simulink model "tracked_robot"  (R2023a)
settings: Solver=FixedStepDiscrete  StartTime=0.0  StopTime=sim_param.t_end  FixedStep=sim_param.dt  RelTol=1e-3  EnableMultiTasking=on
InitFcn:
  | initfcn
values from neighbouring files (symbols this model uses):
  slip_compensation = 1    [plots.m]    (also in tracked_robot_param.m = 0)
undefined symbols (not defined in the file or in its folder): DiscIntNeverNeededParam, param, path_param, sim_param
libraries: simulink x2
settings Model: PacingRate=0.002500  Creator=david  LastModifiedBy=mfocchi
settings SolverCC: AutoInsertRateTranBlk=on
settings OptimizationCC: DefaultParameterBehavior=Inlined  UseDivisionForNetSlopeComputation=on  GainParamInheritBuiltInType=on  UseFloatMulNetSlope=on  InlineInvariantSignals=on  PassReuseOutputArgsAs=Individual arguments  ZeroExternalMemoryAtStartup=off  ZeroInternalMemoryAtStartup=off  NoFixptDivByZeroProtection=on  EfficientFloat2IntCast=on  LifeSpan=1  OptimizeBlockOrder=speed  DifferentSizesBufferReuse=on  EfficientTunableParamExpr=on
settings DebuggingCC: ParameterTunabilityLossMsg=error  UnderSpecifiedDimensionMsg=warning
settings HardwareCC: ProdLongLongMode=on
settings ModelReferenceCC: ModelReferenceMinAlgLoopOccurrences=on
settings SFSimCC: MATLABDynamicMemAlloc=off
settings RTWCC: Description=Embedded Coder  SystemTargetFile=ert.tlc  TemplateMakefile=ert_default_tmf  TargetLang=C++
settings CodeAppCC: ForceParamTrailComments=on  IgnoreCustomStorageClasses=off  OperatorAnnotations=on  SimulinkDataObjDesc=on  SFDataObjDesc=on  CustomSymbolStrGlobalVar=rt$N$M  CustomSymbolStrType=$N$M  CustomSymbolStrFcn=$N$M$F  CustomSymbolStrMacro=$N$M  InsertBlockDesc=on
settings ERTTargetCC: TargetLangStandard=C++11 (ISO)  GenerateSampleERTMain=on  IncludeMdlTerminateFcn=off  CombineSignalStateStructs=on  CodeInterfacePackaging=C++ class  SupportComplex=off  SupportContinuousTime=on  SupportNonInlinedSFcns=on  SupportVariableSizeSignals=on  InlinedParameterPlacement=NonHierarchical  RootIOFormat=Structure reference  ERTCustomFileTemplate=example_file_process.tlc  ERTFilePackagingFormat=CompactWithDataFile

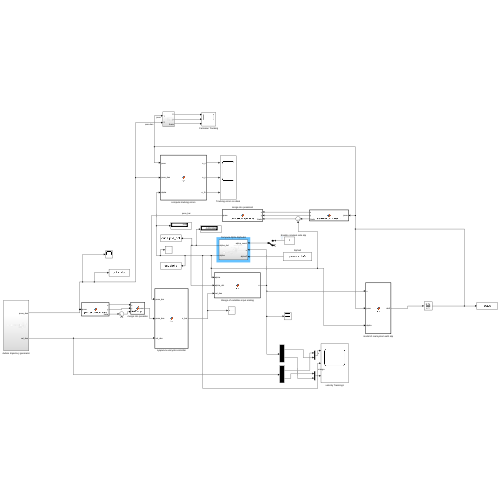
[thumbnail: Simulink's stored preview of the top-level diagram]
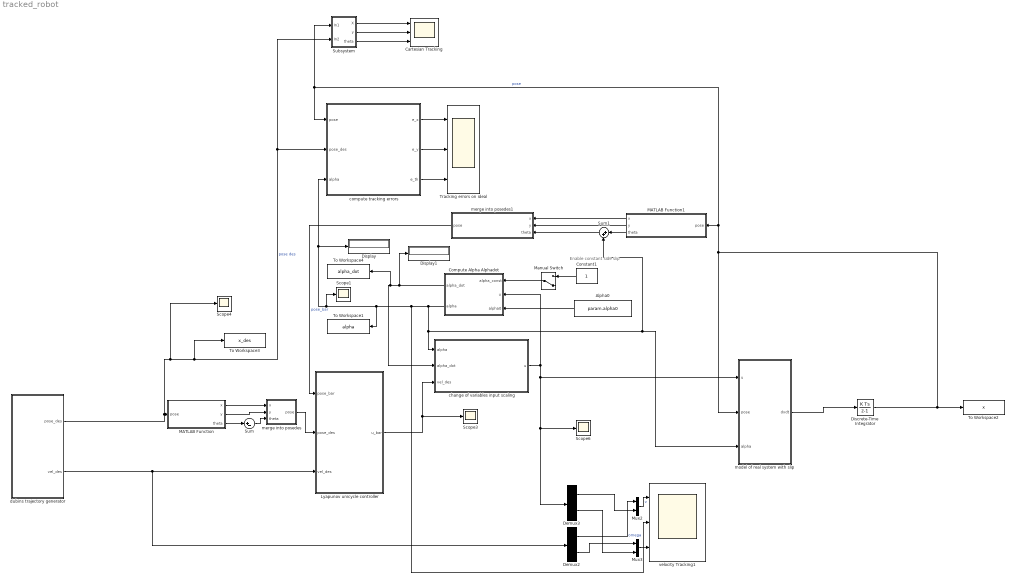
== system tracked_robot ==
  note: Enable constant side slip
  Alpha0 : Constant  Value=param.alpha0
  Cartesian Tracking : Scope  NumInputPorts=3
  Compute Alpha Alphadot : Subsystem
  Constant1 : Constant
  Demux2 : Demux  Outputs=2
  Demux3 : Demux  Outputs=2
  Discrete-Time Integrator : DiscreteIntegrator  InitialCondition=sim_param.initial_state  SampleTime=sim_param.dt  ICPrevOutput=DiscIntNeverNeededParam  ICPrevScaledInput=DiscIntNeverNeededParam
  Display : Display
  Display1 : Display
  Lyapunov unicycle controller : MATLAB Function  TreatAsAtomicUnit=on
  MATLAB Function : MATLAB Function  TreatAsAtomicUnit=on
  MATLAB Function1 : MATLAB Function  TreatAsAtomicUnit=on
  Manual Switch : ManualSwitch  CurrentSetting=0
  Mux2 : Mux  Inputs=2
  Mux3 : Mux  Inputs=2
  Scope{1,3..4,6} (4 alike) : Scope
  Subsystem : Subsystem
  Sum : Sum  Inputs=|+-
  Sum1 : Sum  Inputs=|++
  To Workspace1 : ToWorkspace  VariableName=alpha  SaveFormat=Timeseries  SampleTime=-1
      settings: Decimation=sim_param.decimation
  To Workspace2 : ToWorkspace  VariableName=x  SaveFormat=Timeseries  SampleTime=-1
      settings: Decimation=sim_param.decimation
  To Workspace3 : ToWorkspace  VariableName=x_des  SaveFormat=Timeseries  SampleTime=-1
      settings: Decimation=sim_param.decimation
  To Workspace4 : ToWorkspace  VariableName=alpha_dot  SaveFormat=Timeseries  SampleTime=-1
      settings: Decimation=sim_param.decimation
  Tracking errors on ideal : Scope  NumInputPorts=3
  change of variables input scaling : MATLAB Function  TreatAsAtomicUnit=on
  compute tracking errors : MATLAB Function  TreatAsAtomicUnit=on
  dubins trajectory generator : Subsystem
  merge into posedes : MATLAB Function  TreatAsAtomicUnit=on
  merge into posedes1 : MATLAB Function  TreatAsAtomicUnit=on
  model of real system with slip : MATLAB Function  TreatAsAtomicUnit=on
  velocity Tracking1 : Scope  NumInputPorts=3
  wires:
  model of real system with slip/1(dxdt) -> Discrete-Time Integrator/1
  dubins trajectory generator/1(pose_des) -> Subsystem/2(In2), compute tracking errors/2(pose_des), To Workspace3/1, Scope4/1, MATLAB Function/1(pose)  "pose des"
  Discrete-Time Integrator/1 -> To Workspace2/1, MATLAB Function1/1(pose), Subsystem/1(In1), compute tracking errors/1(pose), model of real system with slip/2(pose)  "pose"
  Lyapunov unicycle controller/1(u_bar) -> Scope3/1, change of variables input scaling/3(vel_des)
  MATLAB Function/1(x) -> merge into posedes/1(x)
  MATLAB Function/2(y) -> merge into posedes/2(y)
  MATLAB Function/3(theta) -> Sum/1
  Sum/1 -> merge into posedes/3(theta)
  merge into posedes/1(pose) -> Lyapunov unicycle controller/2(pose_des)
  compute tracking errors/1(e_x) -> Tracking errors on ideal/1
  compute tracking errors/2(e_y) -> Tracking errors on ideal/2
  compute tracking errors/3(e_th) -> Tracking errors on ideal/3
  Alpha0/1 -> Compute Alpha Alphadot/3(alpha0)
  Compute Alpha Alphadot/1(alpha_dot) -> To Workspace4/1, change of variables input scaling/2(alpha_dot), Display1/1
  Mux2/1 -> velocity Tracking1/1  "v"
  Mux3/1 -> velocity Tracking1/2  "omega"
  dubins trajectory generator/2(vel_des) -> Demux2/1, Lyapunov unicycle controller/3(vel_des)
  Demux2/1 -> Mux2/1
  Demux2/2 -> Mux3/1
  Demux3/1 -> Mux2/2
  Demux3/2 -> Mux3/2
  Constant1/1 -> Manual Switch/1
  Manual Switch/1 -> Compute Alpha Alphadot/1(alpha_const)
  MATLAB Function1/1(x) -> merge into posedes1/1(x)
  MATLAB Function1/2(y) -> merge into posedes1/2(y)
  Sum1/1 -> merge into posedes1/3(theta)
  MATLAB Function1/3(theta) -> Sum1/1
  merge into posedes1/1(pose) -> Lyapunov unicycle controller/1(pose_bar)  "pose_bar"
  Subsystem/1(X) -> Cartesian Tracking/1
  Subsystem/2(y) -> Cartesian Tracking/2
  Subsystem/3(theta) -> Cartesian Tracking/3
  change of variables input scaling/1(u) -> Compute Alpha Alphadot/2(u), Demux3/1, Scope6/1, model of real system with slip/1(u)
  Compute Alpha Alphadot/2(alpha) -> change of variables input scaling/1(alpha), model of real system with slip/3(alpha), Sum1/2, To Workspace1/1, Scope1/1, compute tracking errors/3(alpha), Display/1, velocity Tracking1/3

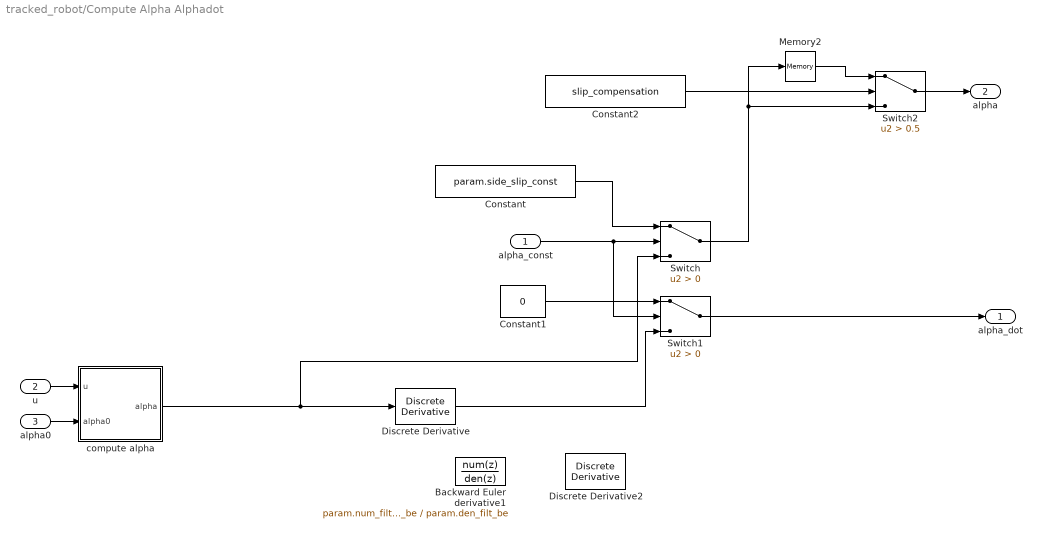
== system tracked_robot/Compute Alpha Alphadot ==
  alpha_const : Inport
  u : Inport  Port=2
  alpha0 : Inport  Port=3
  Backward Euler derivative1 : DiscreteTransferFcn  Numerator=param.num_filt_be  Denominator=param.den_filt_be  InitialStates=1  SampleTime=sim_param.dt
  Constant : Constant  Value=param.side_slip_const
  Constant1 : Constant  Value=0
  Constant2 : Constant  Value=slip_compensation
  Discrete Derivative : simulink/Discrete/Discrete Derivative  gainval=1.0  ICPrevScaledInput=0.0  OutMin=[]  OutMax=[]  OutDataType=fixdt(1, 16)  OutScaling=2^-10  DoSatur=off
  Discrete Derivative2 : simulink/Discrete/Discrete Derivative  gainval=1.0  ICPrevScaledInput=0.0  OutMin=[]  OutMax=[]  OutDataType=fixdt(1, 16)  OutScaling=2^-10  DoSatur=off
  Memory2 : Memory
  Switch : Switch  Criteria=u2 > Threshold  SaturateOnIntegerOverflow=off  InputSameDT=off
  Switch1 : Switch  Criteria=u2 > Threshold  SaturateOnIntegerOverflow=off  InputSameDT=off
  Switch2 : Switch  Criteria=u2 > Threshold  Threshold=0.5  SaturateOnIntegerOverflow=off  InputSameDT=off
  compute alpha : MATLAB Function  TreatAsAtomicUnit=on
  alpha_dot : Outport
  alpha : Outport  Port=2
  wires:
  alpha0/1 -> compute alpha/2(alpha0)
  u/1 -> compute alpha/1(u)
  compute alpha/1(alpha) -> Discrete Derivative/1, Switch/3
  Constant/1 -> Switch/1
  alpha_const/1 -> Switch1/2, Switch/2
  Constant1/1 -> Switch1/1
  Discrete Derivative/1 -> Switch1/3
  Switch1/1 -> alpha_dot/1
  Constant2/1 -> Switch2/2
  Switch/1 -> Switch2/3, Memory2/1
  Memory2/1 -> Switch2/1
  Switch2/1 -> alpha/1

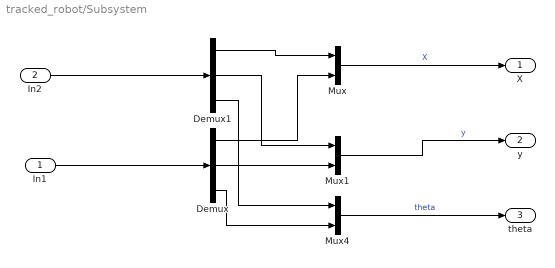
== system tracked_robot/Subsystem ==
  In1 : Inport
  In2 : Inport  Port=2
  Demux : Demux  Outputs=3
  Demux1 : Demux  Outputs=3
  Mux : Mux  Inputs=2
  Mux1 : Mux  Inputs=2
  Mux4 : Mux  Inputs=2
  X : Outport
  y : Outport  Port=2
  theta : Outport  Port=3
  wires:
  Demux1/1 -> Mux/1
  Demux/1 -> Mux/2
  Mux1/1 -> y/1  "y"
  Demux1/2 -> Mux1/1
  Demux1/3 -> Mux4/1
  In1/1 -> Demux/1
  Demux/3 -> Mux4/2
  Mux/1 -> X/1  "X"
  Demux/2 -> Mux1/2
  Mux4/1 -> theta/1  "theta"
  In2/1 -> Demux1/1

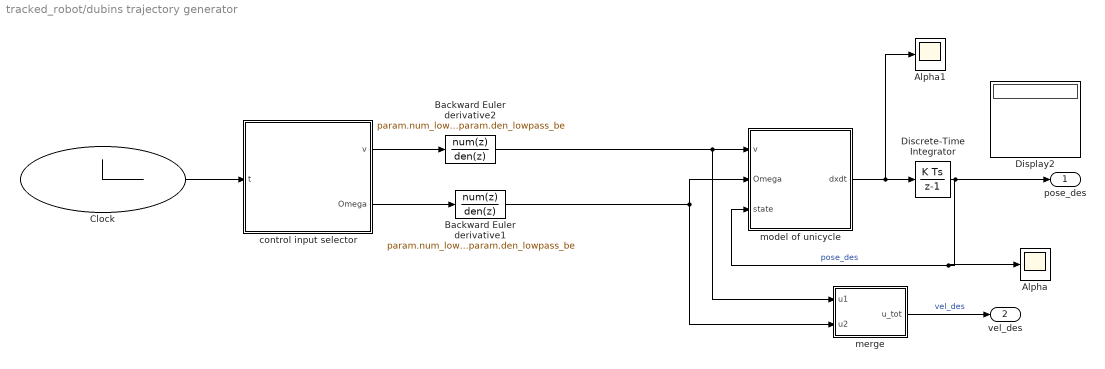
== system tracked_robot/dubins trajectory generator ==
  Alpha : Scope
  Alpha1 : Scope
  Backward Euler derivative1 : DiscreteTransferFcn  Numerator=param.num_lowpass_be  Denominator=param.den_lowpass_be  InitialStates=1  SampleTime=sim_param.dt
  Backward Euler derivative2 : DiscreteTransferFcn  Numerator=param.num_lowpass_be  Denominator=param.den_lowpass_be  InitialStates=1  SampleTime=sim_param.dt
  Clock : Clock
  Discrete-Time Integrator : DiscreteIntegrator  InitialCondition=path_param.init_pose  SampleTime=sim_param.dt  ICPrevOutput=DiscIntNeverNeededParam  ICPrevScaledInput=DiscIntNeverNeededParam
  Display2 : Display
  control input selector : MATLAB Function  TreatAsAtomicUnit=on
  merge : MATLAB Function  TreatAsAtomicUnit=on
  model of unicycle : MATLAB Function  TreatAsAtomicUnit=on
  pose_des : Outport
  vel_des : Outport  Port=2
  wires:
  Discrete-Time Integrator/1 -> Alpha/1, model of unicycle/3(state), pose_des/1  "pose_des"
  merge/1(u_tot) -> vel_des/1  "vel_des"
  control input selector/1(v) -> Backward Euler derivative2/1
  control input selector/2(Omega) -> Backward Euler derivative1/1
  Clock/1 -> control input selector/1(t)
  model of unicycle/1(dxdt) -> Alpha1/1, Discrete-Time Integrator/1
  Backward Euler derivative1/1 -> merge/2(u2), model of unicycle/2(Omega)
  Backward Euler derivative2/1 -> merge/1(u1), model of unicycle/1(v)

== matlab function tracked_robot/dubins trajectory generator/model of unicycle ==
  data: v input; Omega input; dxdt output; state input
function dxdt = fcn(v, Omega, state)

    theta = state(3);
    
    dxdt = [v*cos(theta) , v*sin(theta), Omega];
   

end

== matlab function tracked_robot/Compute Alpha Alphadot/compute alpha ==
  data: u input size=2; alpha0 input size=1; alpha output size=1
function alpha = fcn(u, alpha0)
    v = u(1);
    omega = u(2);
    %alpha = alpha0*omega^2/((v+0.0001)^2);
  
    if (omega == 0)
        turning_radius = 0;
    else 
        turning_radius = v/omega;
    end
    % model side slip as a plyinomial in the curvature
	K = 1/(turning_radius+0.00001);
	alpha = -0.0610487 + (-0.0185)*K +  (-0.0014)*(K*K); % simplified notation
	% alpha = a0 + a1*pow((a2 + 1/R), 2); // original

	if turning_radius < 0.0 
        % turning right		
		 alpha=alpha*(-1);
    end
   %     alpha = -sign(omega)*alpha0*omega^2/((v)^2);
    

end

== matlab function tracked_robot/MATLAB Function1 ==
  data: x output; pose input; y output; theta output
function [x,y,theta] = getPoseComponents(pose)
x = pose(1);
y = pose(2);
theta = pose(3);

== matlab function tracked_robot/merge into posedes1 ==
  data: pose output; x input; y input; theta input
function pose = getPoseComponents(x,y,theta)
pose = [x,y,theta];

== matlab function tracked_robot/dubins trajectory generator/control input selector ==
  data: t input; v output double size=1; Omega output double size=1; path_param parameter
function [v,Omega] = fcn(t, path_param)
    % select the right control input in function of the current time. In
    % the params 5 vectors must be defined:
    % time_vec : list of n times [t1... tn]
    % 

    idx = find(t >= path_param.time_vec, 1, 'last');
    idx = idx(1);
    if(idx >= length(path_param.linear_velocity.q))
        idx = length(path_param.linear_velocity.q);
    end
    vq = path_param.linear_velocity.q(idx);
    vm = path_param.linear_velocity.m(idx);
    aq = path_param.angular_velocity.q(idx);
    am =  path_param.angular_velocity.m(idx);
    
    v     = vm*t + vq;
    Omega = am*t + aq;
end

== matlab function tracked_robot/model of real system with slip ==
  data: u input; dxdt output; pose input; alpha input
function dxdt = fcn(u, pose, alpha)

    theta = pose(3);
    
    v     = u(1);
    Omega = u(2);

    dxdt = [v*cos(theta + alpha) / cos(alpha), v*sin(theta + alpha) / cos(alpha), Omega];
   
end

== matlab function tracked_robot/Lyapunov unicycle controller ==
  data: pose_bar input; pose_des input; u_bar output size=[1,2]; vel_des input; ctrl_param parameter
function u_bar = fcn(pose_bar, pose_des, vel_des, ctrl_param)
    % compute the control for a unicycle using Lyapunov theory
    u_bar = zeros(1,2);

    theta_des = pose_des(3);
    theta_bar = pose_bar(3);

 
 
    if ctrl_param.controller_type == 1

        error_x     = pose_bar(1) - pose_des(1);
        error_y     = pose_bar(2) - pose_des(2);
        error_theta = theta_bar - theta_des;

        V_hat = vel_des(1);
        Omega_hat = vel_des(2);
    
        Kp = ctrl_param.Kp;
        K_theta = ctrl_param.K_theta;
    
        psi = atan2(error_y, error_x);
        alpha = (theta_bar + theta_des) / 2.0;
        error_xy = sqrt(error_x^2 + error_y^2);
    
    
        dv = - Kp * error_xy * cos(theta_bar - psi);
        domega =  - K_theta * error_theta - V_hat * sinc(error_theta / (2)) * error_xy * sin(psi - alpha);
    
        u_bar(1) = V_hat + dv;
        u_bar(2) = Omega_hat + domega;
    
    
    
    elseif ctrl_param.controller_type == 2
    
        error_x     = pose_des(1) - pose_bar(1);
        error_y     = pose_des(2) - pose_bar(2);
        error_theta = theta_des - theta_bar;
        % Kanayama controller (not polar variables) we consider both ex and ey
        % separately!
        V_d= vel_des(1);
        Omega_d = vel_des(2);
    
        Kx = ctrl_param.Kp;
        K_theta = ctrl_param.K_theta;
    
        %express errors in the base frame
        base_error_x     = cos(theta_bar) * error_x + sin(theta_bar)*error_y;
        base_error_y     = -sin(theta_bar) *error_x + cos(theta_bar)*error_y;
    
        %command velocity
        u_bar(1) = V_d*cos(error_theta) + Kx*base_error_x;
        u_bar(2) = Omega_d + K_theta*sin(error_theta) + V_d*base_error_y;
    
    else
        disp('wrong controller')
    end



end

== matlab function tracked_robot/merge into posedes ==
  data: pose output; x input; y input; theta input
function pose = getPoseComponents(x,y,theta)
pose = [x,y,theta];

== matlab function tracked_robot/MATLAB Function ==
  data: x output; pose input; y output; theta output
function [x,y,theta] = getPoseComponents(pose)
x = pose(1);
y = pose(2);
theta = pose(3);

== matlab function tracked_robot/change of variables input scaling ==
  data: alpha input; alpha_dot input; u output size=[1,2]; vel_des input; slip_compensation parameter
function u = fcn(alpha, alpha_dot,vel_des, slip_compensation)
    u = zeros(1,2);

    v_bar = vel_des(1);
    Omega_bar = vel_des(2);
       

   if (slip_compensation == 0) 
        u = vel_des;
   else
        u(1) = v_bar * cos(alpha); 
        u(2) = Omega_bar - alpha_dot;
   end
end

== matlab function tracked_robot/dubins trajectory generator/merge ==
  data: u1 input; u_tot output; u2 input
function u_tot = fcn(u1,u2)
    u_tot = [u1,u2];
end

== matlab function tracked_robot/compute tracking errors ==
  data: pose input; pose_des input; alpha input; e_x output; e_y output; e_th output
function [e_x,e_y, e_th] = fcn(pose, pose_des, alpha)
    % compute the tracking errors with respect to the reference input. Note that the
    % orientation error is not the one of the robot but takes into account
    % the side slip angle.

    theta_des = pose_des(3);
    theta = pose(3);

    e_x = pose(1)-pose_des(1);
    e_y = pose(2)-pose_des(2);
    e_th = (theta+alpha)  - theta_des; % whenever the compensation does its job theta_bar converges to theta+alpha so we need to check if theta+alpha converges to theta_des
                                       % if you want theta converging to
                                       % correct orient theta des then you need to
                                       % add an offset alpha to theta des
                                       
end
